simulink model "Rectificador_Tarea"  (R2024b)
settings: Solver=VariableStepAuto  StartTime=0.0  StopTime=0.1  RelTol=1e-3

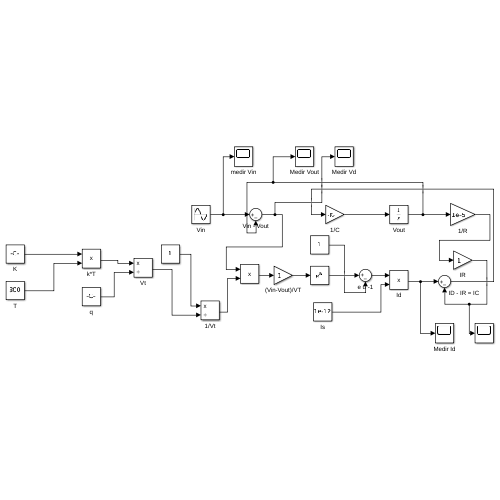
[thumbnail: Simulink's stored preview of the top-level diagram]
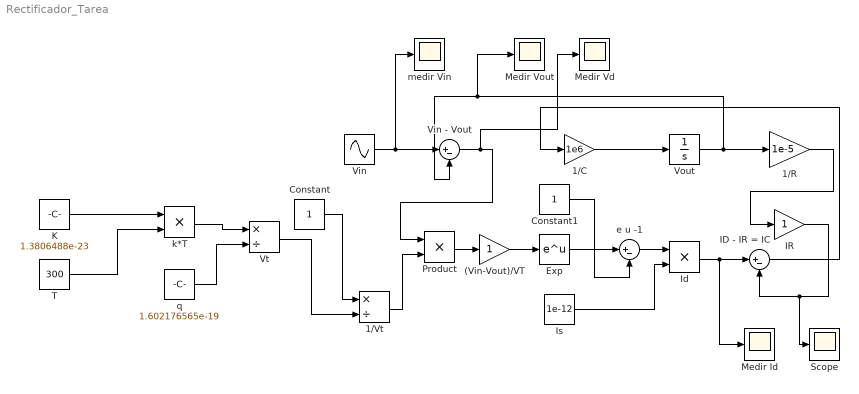
== system Rectificador_Tarea ==
  "                       ID - IR = IC" : Sum  Inputs=|+-
  (Vin-Vout)/VT : Gain
  1/C : Gain  Gain=1e6
  1/R : Gain  Gain=1e-5
  1/Vt : Product  Inputs=*/
  Constant : Constant
  Constant1 : Constant
  Exp : Math
  IR : Gain
  Id : Product
  Is : Constant  Value=1e-12
  K : Constant  Value=1.3806488e-23
  Medir Id : Scope
  Medir Vd : Scope
  Medir Vout : Scope
  Product : Product
  Scope : Scope
  T : Constant  Value=300
  Vin : Sin  Amplitude=12  Frequency=2*pi*60  SampleTime=0
  Vin - Vout : Sum  Inputs=|+-
  Vout : Integrator
  Vt : Product  Inputs=*/
  e u -1 : Sum  Inputs=|+-
  k*T : Product
  medir Vin : Scope
  q : Constant  Value=1.602176565e-19
  wires:
  K/1 -> k*T/1
  T/1 -> k*T/2
  k*T/1 -> Vt/1
  q/1 -> Vt/2
  Vin/1 -> medir Vin/1, Vin - Vout/1
  Constant/1 -> 1/Vt/1
  Vt/1 -> 1/Vt/2
  Vin - Vout/1 -> Medir Vd/1, Product/1
  1/Vt/1 -> Product/2
  Product/1 -> (Vin-Vout)/VT/1
  (Vin-Vout)/VT/1 -> Exp/1
  Constant1/1 -> e u -1/2
  Exp/1 -> e u -1/1
  e u -1/1 -> Id/1
  Is/1 -> Id/2
  1/C/1 -> Vout/1
  1/R/1 -> IR/1
  Id/1 -> Medir Id/1, "                       ID - IR = IC"/1
  IR/1 -> Scope/1, "                       ID - IR = IC"/2
  "                       ID - IR = IC"/1 -> 1/C/1
  Vout/1 -> 1/R/1, Medir Vout/1, Vin - Vout/2
